simulink model "RollCommand"  (R2012b)
settings: configuration reference "configSetObj_autopilot" (kept outside this file)
settings Model: RequirementInfo={} %GIDa_02569d69_523d_4b8c_a66c_0f8416bbb5b9  Creator=ssauvage  LastModifiedBy=ssauvage

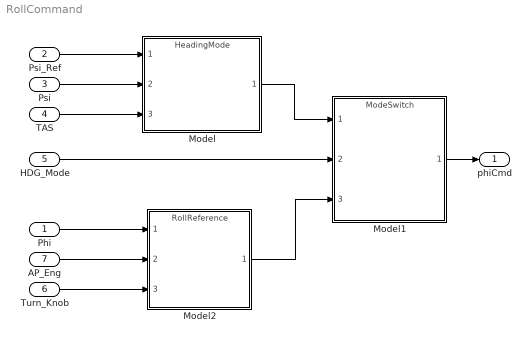
== system RollCommand ==
  Phi : Inport  RequirementInfo={} %GIDa_8c20552a_74b0_4595_97f8_a71e9d0437df  OutDataTypeStr=double
  Psi_Ref : Inport  RequirementInfo={} %GIDa_3b7f6c3b_7df5_4e58_a478_170b04d4dd91  Port=2  OutDataTypeStr=double
  Psi : Inport  RequirementInfo={} %GIDa_97093342_6768_4bec_9372_52bd65a1e7e0  Port=3  OutDataTypeStr=double
  TAS : Inport  RequirementInfo={} %GIDa_18f89cd0_dd21_4908_ae9d_70a9fd70a73d  Port=4  OutDataTypeStr=double
  HDG_Mode : Inport  RequirementInfo={} %GIDa_7e1b19a1_b80e_4970_add0_87f7d2376eb4  Port=5  OutDataTypeStr=boolean
  Turn_Knob : Inport  RequirementInfo={} %GIDa_82f12caf_4270_4b54_afe3_2430658d1f02  Port=6  OutDataTypeStr=double
  AP_Eng : Inport  RequirementInfo={} %GIDa_28443cab_1710_41ec_8440_5a791f19877b  Port=7  OutDataTypeStr=boolean
  Model : ModelReference  RequirementInfo={} %GIDa_28164aa3_a997_4a79_bdf6_0bea9082bf99  ModelNameDialog=HeadingMode  SimulationMode=Normal  ModelReferenceVersion=1.7  CopyOfModelName=HeadingMode  DefaultDataLogging=on
  Model1 : ModelReference  RequirementInfo={} %GIDa_2170bcf7_d9c9_44e3_950f_01d5ad40e849  ModelNameDialog=ModeSwitch  SimulationMode=Normal  ModelReferenceVersion=1.5  CopyOfModelName=ModeSwitch  DefaultDataLogging=on
  Model2 : ModelReference  RequirementInfo={} %GIDa_9c69968a_4938_408e_9e30_87ce9f6e9976  ModelNameDialog=RollReference  SimulationMode=Normal  ModelReferenceVersion=1.16  CopyOfModelName=RollReference  DefaultDataLogging=on
  phiCmd : Outport  RequirementInfo={} %GIDa_eceb2687_af99_40ab_9a00_212ead3a4cd9
  wires:
  Model/1 -> Model1/1
  Model2/1 -> Model1/3
  Psi_Ref/1 -> Model/1
  Psi/1 -> Model/2
  TAS/1 -> Model/3
  HDG_Mode/1 -> Model1/2
  Model1/1 -> phiCmd/1
  Phi/1 -> Model2/1
  AP_Eng/1 -> Model2/2
  Turn_Knob/1 -> Model2/3
